simulink model "MicroFSMPCCLACPU1"  (R2024a)
settings: Solver=FixedStepAuto  StartTime=0.0  StopTime=Inf  RelTol=1e-3  EnableMultiTasking=on
values from neighbouring files (symbols this model uses):
  ar = single(round(1/10,3))    [Para_Motor_Micro.m]
  PI_params = mcb.internal.SetControllerParameters(pmsm,inverter,SI_System,T_pwm,Ts,Ts_speed)    [Para_Motor_Micro.m]
  Tabf = round(Tab',3)    [Para_Motor_Micro.m]
  target = mcb_SetProcessorDetails('F28379D',PWM_frequency)    [Para_Motor_Micro.m]
  Ts = T_pwm    (= 3e-05)    [Para_Motor_Micro.m]
  Ts_com = 2*1*Ts    (= 6e-05)    [Para_Motor_Micro.m]
undefined symbols (not defined in the file or in its folder): C28x, codertarget, CPU1, CPU2, Down, dyV, gmax, GPTRIP1SEL, GPTRIP2SEL, inverter, Ls, PWM_Counter_PeriodVel, R, Tab, Tv, Tvz, TZ1, TZ2, ud, Up
libraries: mcbcontrolslib x28, c2802xlib x18, c2837xDlib x13, dsparch4 x6, eeTransforms x5, slpidlib x4, mcbpositiondecoderlib x3, simulink x2, c2806xlib x1, spsabctoAlphaBetaZeroLib x1, c280xlib x1, c2000lib x1
(part 6 of 8)

== matlab function MicroFSMPCCLACPU1/ADC-PWM /Control_System/Closed Loop Control/FS-MPC Sobre muestreo modulado ==
  settings: updateMethod=DISCRETE
  data: I input; Gate output size=3; FEM input size=2; iAref input; iBref input; mode input; Vbus input; J output size=1

function [Gate,J]      = fcn(I,FEM,iAref,iBref,mode,Vbus)


%%%%%Init Parameters%%%%%%%
Ts=single(3.2e-5);
R=single(1) ;
L=single(2.00e-3);
M=(3/7)*L;
Ls=single(L+M);
ud=single(170);
%alphe=single(0.5);
gmax=single(10000);
n=single(3);
moder=mode;

% uAnull=single(0);
% uBnull=single(0);
Div=single(4); %%%%Numero de divisiones 
dy0=single(0.12);
dyV=(1-dy0)/Div;
Tv=dyV*Ts;
Tvz=Ts*(dy0/2+dyV);
%Tp=single(Ts*0.9);
 persistent     Gates Gop jop iA1o iB1o Gop1 jop1 iA2o iB2o Gop2 jop2 Gop3 jop3 iA3o iB3o status1  %tick status1 
  if isempty(Gates)
        Gates=single([0,0,0]');

        Gop=gmax;
        jop=single(1);
        iA1o=single(0);
        iB1o=single(0);

        Gop1=gmax;
        jop1=single(1);
        iA2o=single(0);
        iB2o=single(0);

        Gop2=gmax;
        jop2=single(1);
        iA3o=single(0);
        iB3o=single(0);

        Gop3=gmax;
        jop3=single(1);

     end


%%%%%%Read mesurments%%%%%%%%%%%%
%ud=single(Vbus);
iA=I(1);
iB=I(2);
eA=FEM(1);
eB=FEM(2);

% eA1=FEM1(1);
% eB1=FEM1(2);
% fa=eA/(Ke*w);
% fb=eB/(Ke*w);
% fa1=fa;
% fb1=fb;
% ua=u(1);
% ub=u(2);



 % % %%%7 vectores ordenados ab separados flotando
%  status1=[0,1,0,1,0,1	;
%      1,0,0,0,0,1	;
%  0,0,1,0,0,1	;
%  0,1,1,0,0,0	;
%  0,1,0,0,1,0	;
%  0,0,0,1,1,0	;
%  1,0,0,1,0,0	;];
% 
%  u1=ud*[0	,	0	;
%      1/2	,	sqrt(3)/6 	;
% 0	,	sqrt(3)/3	;
% -1/2	,	sqrt(3)/6 	;
% -1/2	,	-sqrt(3)/6 	;
% 0	,	-sqrt(3)/3	;
% 1/2	,	-sqrt(3)/6 	;
% ];

%%%%%%For loop 3%%%%%%      
% %%%7 vectores ordenados ab tradicionales
%  status1=[1,1,1;
%           1,0,0	;
%           1,1,0;
%           0,1,0;
%            0,1,1	;
%            0,0,1	;
%            1,0,1;
%            ];
% % 
%  u1=ud*[0	,	0	;
%       2/3	,	0	;
%       1/3	,	1/sqrt(3)	;%parece estar aml el vector
%   -1/3	,	1/sqrt(3)	;
%  -2/3	,	0	;
%  -1/3	,	-1/sqrt(3)	;
%   1/3	,	-1/sqrt(3)	;
%   ];


 if mode==1
  u1=ud*[0	,	0	;
2/3	,	0	;
1/3	,	1/sqrt(3)];
elseif mode==2
 
 u1=ud*[0	,	0	;
1/3	,	1/sqrt(3)	;
-1/3	,	1/sqrt(3)	;];   
elseif mode==3

 u1=ud*[0	,	0	;
-1/3	,	1/sqrt(3)	;
-2/3	,	0	;];  
 elseif mode==4
 
 u1=ud*[0	,	0	;
-2/3	,	0	;
-1/3	,	-1/sqrt(3)	;];
 elseif mode==5
  
 u1=ud*[0	,	0	;
-1/3	,	-1/sqrt(3)	;
1/3	,	-1/sqrt(3)	;];
 elseif mode==6
  
 u1=ud*[0	,	0	;
1/3	,	-1/sqrt(3)	;
2/3	,	0	;];

else
   
 u1=ud*[0	,	0	;
2/3	,	0	;
1/3	,	1/sqrt(3)]; 
end

%%%%%%%%FSMPC%%%%%%%%%%%%%%%%%%%%%%%%%%%%%%%%%%%%%

      Gop=gmax;
      jop=single(1);
      Gop1=gmax;
      jop1=single(1);
      Gop2=gmax;
      jop2=single(1);
      Gop3=gmax;
      jop3=single(1);

%%%%%%For n loop N1  %%%%%% 
     for j= 1:n    
  uA1=u1(j,1);
  uB1=u1(j,2);

%%%%%%For loop 3 combinacion de vectores 1%%%%%% 
     iA1= iA + (1/Ls)*(Tv*uA1)- (Tvz/Ls)*(eA+R*iA);
     iB1=iB + (1/Ls)*(Tv*uB1)- (Tvz/Ls)*(eB+R*iB);
     
     G=(iAref-iA1)^2+(iBref-iB1)^2 ; 

          if G<Gop
          Gop=G;
          jop=j;
          iA1o=iA1;
          iB1o=iB1;
   
          end
     end

 %%%%%%For n loop N2  %%%%%% 
  for j1= 1:n    
  uA1=u1(j1,1);
  uB1=u1(j1,2);

%%%%%%For loop 3 combinacion de vectores 1%%%%%% 
     iA1= iA1o + (1/Ls)*(Tv*uA1)- (Tv/Ls)*(eA+R*iA1o);
     iB1=iB1o + (1/Ls)*(Tv*uB1)- (Tv/Ls)*(eB+R*iB1o);
     
     G=(iAref-iA1)^2+(iBref-iB1)^2 ; 

          if G<Gop
          Gop1=G;
          jop1=j1;
          iA2o=iA1;
          iB2o=iB1;
   
          end
  end    


 %%%%%%For n loop N3  %%%%%% 
  for j2= 1:n    
  uA1=u1(j2,1);
  uB1=u1(j2,2);

%%%%%%For loop 3 combinacion de vectores 1%%%%%% 
     iA1= iA2o + (1/Ls)*(Tv*uA1)- (Tv/Ls)*(eA+R*iA2o);
     iB1=iB2o + (1/Ls)*(Tv*uB1)- (Tv/Ls)*(eB+R*iB2o);
     
     G=(iAref-iA1)^2+(iBref-iB1)^2 ; 

          if G<Gop
          Gop2=G;
          jop2=j2;
          iA3o=iA1;
          iB3o=iB1;
   
          end
  end   
  

 %%%%%%For n loop N4  %%%%%% 
  for j3= 1:n    
  uA1=u1(j3,1);
  uB1=u1(j3,2);

%%%%%%For loop 3 combinacion de vectores 1%%%%%% 
     iA1= iA3o + (1/Ls)*(Tv*uA1)- (Tvz/Ls)*(eA+R*iA3o);
     iB1=iB3o + (1/Ls)*(Tv*uB1)- (Tvz/Ls)*(eB+R*iB3o);
     
     G=(iAref-iA1)^2+(iBref-iB1)^2 ; 

          if G<Gop
          Gop3=G;
          jop3=j3;
      
   
          end
  end   

    
%%%%Apply conmutation states%%%%%%%%%%%%%%%%%%%%%%%  


   % Gates=status1(jop,:)';

%To=dyV*((indexv(1,jop)==1)+(indexv(2,jop)==1)+(indexv(3,jop)==1)+(indexv(4,jop)==1))+dy0;
%To=0;
% Ta=dyV*((indexv(1,jop)==2)+(indexv(2,jop)==2)+(indexv(3,jop)==2)+(indexv(4,jop)==2));
% Tb=dyV*((indexv(1,jop)==3)+(indexv(2,jop)==3)+(indexv(3,jop)==3)+(indexv(4,jop)==3));
Ta=dyV*((jop==2)+(jop1==2)+(jop2==2)+(jop3==2));
Tb=dyV*((jop==3)+(jop1==3)+(jop2==3)+(jop3==3));

  TA=(moder==1)*(Tb+Ta)+(moder==6)*(Tb+Ta)+(moder==2)*(Ta)+(moder==5)*(Tb);
  TB=(moder==1)*(Tb)+(moder==2)*(Tb+Ta)+(moder==3)*(Tb+Ta)+(moder==4)*(Ta);
  TC=(moder==6)*(Ta)+(moder==3)*(Tb)+(moder==4)*(Tb+Ta)+(moder==5)*(Tb+Ta);




% TA=(moder==6)*(To+Tb+Ta)+(moder==5)*(To+Tb+Ta)+(moder==1)*(To+Ta)+(moder==2)*(To)+(moder==3)*(To)+(moder==4)*(To+Tb);
% TB=(moder==5)*(To)+(moder==6)*(To+Tb)+(moder==1)*(To+Tb+Ta)+(moder==2)*(To+Tb+Ta)+(moder==3)*(To+Ta)+(moder==4)*(To);
% TC=(moder==5)*(To+Ta)+(moder==6)*(To)+(moder==1)*(To)+(moder==2)*(To+Tb)+(moder==3)*(To+Tb+Ta)+(moder==4)*(To+Tb+Ta);

Gates=[TA,TB,TC]';
J=jop;
Gate=Gates;
%tie=t2;
%jl=jn;
%j=1;




%   TA=(moder==1)*(To+Tb+Ta)+(moder==6)*(To+Tb+Ta)+(moder==2)*(To+Ta)+(moder==3)*(To)+(moder==4)*(To)+(moder==5)*(To+Tb);
% % TA=(moder==6)*(To+Tb+Ta)+(moder==5)*(To+Tb+Ta)+(moder==1)*(To+Ta)+(moder==2)*(To)+(moder==3)*(To)+(moder==4)*(To+Tb);
%   TB=(moder==6)*(To)+(moder==1)*(To+Tb)+(moder==2)*(To+Tb+Ta)+(moder==3)*(To+Tb+Ta)+(moder==4)*(To+Ta)+(moder==5)*(To);
% % TB=(moder==5)*(To)+(moder==6)*(To+Tb)+(moder==1)*(To+Tb+Ta)+(moder==2)*(To+Tb+Ta)+(moder==3)*(To+Ta)+(moder==4)*(To);
%   TC=(moder==6)*(To+Ta)+(moder==1)*(To)+(moder==2)*(To)+(moder==3)*(To+Tb)+(moder==4)*(To+Tb+Ta)+(moder==5)*(To+Tb+Ta);

== matlab function MicroFSMPCCLACPU1/ADC-PWM /Control_System/Closed Loop Control/FS-MPC Sobre muestreo modulado clean ==
  settings: updateMethod=DISCRETE
  data: I input; Gate output size=3; FEM input size=2; iAref input; iBref input; mode input; J output size=1; Ts parameter; R parameter; Ls parameter; ud parameter; gmax parameter; Tv parameter; Tvz parameter; dyV parameter

function [Gate, J]      = fcn(I,FEM,iAref,iBref,mode,Ts, R, Ls, ud, gmax, Tv, Tvz, dyV)


%%%%%Init Parameters%%%%%%%
% Ts=single(2.5e-5);
% %Ts=single(5e-5);
% %Ts=single(3.2e-05);
% R=single(1) ;
% %L=single(9.75e-3);
%  L=single(2.02e-3);
% %L=single(1.45e-3);
%   %L=single(Lp);
%   %L=single(1.85e-3);
%  M=(3/7)*L;
% %Lt=(7/3)*M;
% Ls=single(L+M);
% %Ls=single(L);
% %Ls=single(L);
% %ud=240;
% ud=single(170);

%Kt =single(0.3811);
%T0=Ts*(1);
%Ke=single(0.3455);
%gmax=single(100000);
n=single(3);

% % uAnull=single(0);
% % uBnull=single(0);
% Div=single(4); %%%%Numero de divisiones 
% dy0=single(0.1);
% dyV=(1-dy0)/Div;
% Tv=dyV*Ts;
% Tvz=Ts*(dy0/2+dyV);
%Tp=single(Ts*0.9);
 persistent     Gates Gop jop iA1o iB1o Gop1 jop1 iA2o iB2o Gop2 jop2 Gop3 jop3 iA3o iB3o  %tick status1 
  if isempty(Gates)
        Gates=single([0,0,0]');

        Gop=gmax;
        jop=single(1);
        iA1o=single(0);
        iB1o=single(0);

        Gop1=gmax;
        jop1=single(1);
        iA2o=single(0);
        iB2o=single(0);

        Gop2=gmax;
        jop2=single(1);
        iA3o=single(0);
        iB3o=single(0);

        Gop3=gmax;
        jop3=single(1);


     end


%%%%%%Read mesurments%%%%%%%%%%%%
%ud=single(Vbus);

iA=I(1);
iB=I(2);
eA=FEM(1);
eB=FEM(2);
moder=mode;



 if mode==1
 u1=ud*[0	,	0	;
2/3	,	0	;
1/3	,	1/sqrt(3)];
elseif mode==2
 
 u1=ud*[0	,	0	;
1/3	,	1/sqrt(3)	;
-1/3	,	1/sqrt(3)	;];   
elseif mode==3
   
 u1=ud*[0	,	0	;
-1/3	,	1/sqrt(3)	;
-2/3	,	0	;];  
 elseif mode==4
  
 u1=ud*[0	,	0	;
-2/3	,	0	;
-1/3	,	-1/sqrt(3)	;];
 elseif mode==5
   
 u1=ud*[0	,	0	;
-1/3	,	-1/sqrt(3)	;
1/3	,	-1/sqrt(3)	;];
 elseif mode==6
   
 u1=ud*[0	,	0	;
1/3	,	-1/sqrt(3)	;
2/3	,	0	;];

else
 
 u1=ud*[0	,	0	;
2/3	,	0	;
1/3	,	1/sqrt(3)]; 
end

%%%%%%%%FSMPC%%%%%%%%%%%%%%%%%%%%%%%%%%%%%%%%%%%%%

      Gop=gmax;
      jop=single(1);
      Gop1=gmax;
      jop1=single(1);
      Gop2=gmax;
      jop2=single(1);
      Gop3=gmax;
      jop3=single(1);

%%%%%%For n loop N1  %%%%%% 
     for j= 1:n    
  uA1=u1(j,1);
  uB1=u1(j,2);

%%%%%%For loop 3 combinacion de vectores 1%%%%%% 
     iA1= iA + (1/Ls)*(Tv*uA1)- (Tvz/Ls)*(eA+R*iA);
     iB1=iB + (1/Ls)*(Tv*uB1)- (Tvz/Ls)*(eB+R*iB);
     
     G=(iAref-iA1)^2+(iBref-iB1)^2 ; 

          if G<Gop
          Gop=G;
          jop=j;
          iA1o=iA1;
          iB1o=iB1;
   
          end
     end

 %%%%%%For n loop N2  %%%%%% 
  for j1= 1:n    
  uA1=u1(j1,1);
  uB1=u1(j1,2);

%%%%%%For loop 3 combinacion de vectores 1%%%%%% 
     iA1= iA1o + (1/Ls)*(Tv*uA1)- (Tv/Ls)*(eA+R*iA1o);
     iB1=iB1o + (1/Ls)*(Tv*uB1)- (Tv/Ls)*(eB+R*iB1o);
     
     G=(iAref-iA1)^2+(iBref-iB1)^2 ; 

          if G<Gop
          Gop1=G;
          jop1=j1;
          iA2o=iA1;
          iB2o=iB1;
   
          end
  end    


 %%%%%%For n loop N3  %%%%%% 
  for j2= 1:n    
  uA1=u1(j2,1);
  uB1=u1(j2,2);

%%%%%%For loop 3 combinacion de vectores 1%%%%%% 
     iA1= iA2o + (1/Ls)*(Tv*uA1)- (Tv/Ls)*(eA+R*iA2o);
     iB1=iB2o + (1/Ls)*(Tv*uB1)- (Tv/Ls)*(eB+R*iB2o);
     
     G=(iAref-iA1)^2+(iBref-iB1)^2 ; 

          if G<Gop
          Gop2=G;
          jop2=j2;
          iA3o=iA1;
          iB3o=iB1;
   
          end
  end   
  

 %%%%%%For n loop N4  %%%%%% 
  for j3= 1:n    
  uA1=u1(j3,1);
  uB1=u1(j3,2);

%%%%%%For loop 3 combinacion de vectores 1%%%%%% 
     iA1= iA3o + (1/Ls)*(Tv*uA1)- (Tvz/Ls)*(eA+R*iA3o);
     iB1=iB3o + (1/Ls)*(Tv*uB1)- (Tvz/Ls)*(eB+R*iB3o);
     
     G=(iAref-iA1)^2+(iBref-iB1)^2 ; 

          if G<Gop
          Gop3=G;
          jop3=j3;
      
   
          end
  end   

    
%%%%Apply conmutation states%%%%%%%%%%%%%%%%%%%%%%%  


Ta=dyV*((jop==2)+(jop1==2)+(jop2==2)+(jop3==2));
Tb=dyV*((jop==3)+(jop1==3)+(jop2==3)+(jop3==3));

  TA=(moder==1)*(Tb+Ta)+(moder==6)*(Tb+Ta)+(moder==2)*(Ta)+(moder==5)*(Tb);
  TB=(moder==1)*(Tb)+(moder==2)*(Tb+Ta)+(moder==3)*(Tb+Ta)+(moder==4)*(Ta);
  TC=(moder==6)*(Ta)+(moder==3)*(Tb)+(moder==4)*(Tb+Ta)+(moder==5)*(Tb+Ta);


Gates=[TA,TB,TC]';
J=jop;
Gate=Gates;

== matlab function MicroFSMPCCLACPU1/ADC-PWM /Control_System/Closed Loop Control/FS-MPC opt tiempo complex Clean ==
  settings: updateMethod=DISCRETE
  data: I input; Gate output size=3; FEM input size=2; iAref input; iBref input; J output size=1; mode input; moder input

function [Gate,J]      = fcn(I,FEM,iAref,iBref,mode,moder)


%%%%%Init Parameters%%%%%%%
Ts=single(2.5e-5);
R=single(1) ;
L=single(1.85e-3);
M=(3/7)*L;
Ls=single(L+M);
ud=single(170);
alphe=single(0.5);
gmax=single(10000);
n=single(3);
nk=single(3);


 persistent     Gates Gop jop  Trop Tr  status1
  if isempty(Gates)
        Gates=single([0,0,0]');
        Gop=gmax;
        jop=single(1);
        Tr=single(0);
        Trop=single(0);

status1=[
 1,1,0;
 0,1,0;
 0,0,0;]; 
     end


%%%%%%Read mesurments%%%%%%%%%%%%
iA=I(1);
iB=I(2);
eA=FEM(1);
eB=FEM(2);


%%%%Moded
%  if mode==1
%  status1=[0,0,0;
%  1,0,0	;
% 1,1,0;];   
%  u1=ud*[0	,	0	;
% 2/3	,	0	;
% 1/3	,	1/sqrt(3)];
% elseif mode==2
%  status1=[0,0,0;
% 1,1,0	;
% 0,1,0	;];   
%  u1=ud*[0	,	0	;
% 1/3	,	1/sqrt(3)	;
% -1/3	,	1/sqrt(3)	;];   
% elseif mode==3
%  status1=[0,0,0;
% 0,1,0	;
% 0,1,1	;];   
%  u1=ud*[0	,	0	;
% -1/3	,	1/sqrt(3)	;
% -2/3	,	0	;];  
%  elseif mode==4
%  status1=[0,0,0;
%  0,1,1	;
% 0,0,1	;];   
%  u1=ud*[0	,	0	;
% -2/3	,	0	;
% -1/3	,	-1/sqrt(3)	;];
%  elseif mode==5
%  status1=[0,0,0;
%  0,0,1	;
% 1,0,1	;];   
%  u1=ud*[0	,	0	;
% -1/3	,	-1/sqrt(3)	;
% 1/3	,	-1/sqrt(3)	;];
%  elseif mode==6
%  status1=[0,0,0
% 1,0,1	;
%  1,0,0	;];   
%  u1=ud*[0	,	0	;
% 1/3	,	-1/sqrt(3)	;
% 2/3	,	0	;];
% 
% else
%  status1=[0,0,0;
%  1,0,0	;
% 1,1,0;];   
%  u1=ud*[0	,	0	;
% 2/3	,	0	;
% 1/3	,	1/sqrt(3)]; 
% end

%%%13 vectores totales, 12 modes
 if mode==1 %%%%V0,V1,V12
 u1=ud*[2/3	,	0	;
1/2	,	1/(2*sqrt(3));
0	,	0	;];
elseif mode==2 %%%%V0,V12,V2
 u1=ud*[1/2	,	1/(2*sqrt(3))	;
1/3	,	1/sqrt(3);
0	,	0	;];

elseif mode==3
  u1=ud*[1/3	,	1/sqrt(3)	;
0	,	1/sqrt(3)	;
0	,	0	;];   
  elseif mode==4
  u1=ud*[0	,	1/sqrt(3)	;
-1/3	,	1/sqrt(3)	;
0	,	0	;]; 


elseif mode==5
 u1=ud*[-1/3	,	1/sqrt(3)	;
-1/2	,	1/(2*sqrt(3))	;
0	,	0	;];  

elseif mode==6
 u1=ud*[-1/2	,	1/(2*sqrt(3))	;
-2/3	,	0	;
0	,	0	;];  

 elseif mode==7
 u1=ud*[-2/3	,	0	;
-1/2	,	-1/(2*sqrt(3));
0	,	0	;];

  elseif mode==8
 u1=ud*[-1/2	,	-1/(2*sqrt(3))	;
-1/3	,	-1/sqrt(3)	;
0	,	0	;];


 elseif mode==9
 u1=ud*[
-1/3	,	-1/sqrt(3)	;
0	,	-1/sqrt(3)	;
0	,	0	;];

  elseif mode==10
 u1=ud*[
0	,	-1/sqrt(3)	;
1/3	,	-1/sqrt(3)	;
0	,	0	;];


 elseif mode==11
 u1=ud*[
1/3	,	-1/sqrt(3)	;
1/2	,	-1/(2*sqrt(3))	;
0	,	0	;];

  elseif mode==12
 u1=ud*[
1/2	,	-1/(2*sqrt(3))	;
2/3	,	0	;
0	,	0	;];

else
 
 u1=ud*[
2/3	,	0	;
1/3	,	1/sqrt(3);
0	,	0	;]; 
end
%%%%%%%%FSMPC%%%%%%%%%%%%%%%%%%%%%%%%%%%%%%%%%%%%%

      Gop=gmax;
      jop=single(1);
       ar=single(0.9/7);
%%%%%%For n loop N1  %%%%%% 
for p= 1:nk

    if p==1
        n=single(3);
    else
        n=single(2);
    end    
    Tr1=ar*(2*p);

%%%%%%%%%%%%%%%%%%%%%%%%%%%%%%%%%%%%%%%%%%%%%%%%%%
     for j= 1:n    
     uA1=u1((j),1);
     uB1=u1((j),2);
%%%%%%For loop %%%%%%%%%%%%%%%%%%%%%%%%%%%%%%%%% 
     iA1= iA + (1/Ls)*(Tr1*Ts*uA1)- (Ts/Ls)*(eA+R*iA);
     iB1=iB + (1/Ls)*(Tr1*Ts*uB1)- (Ts/Ls)*(eB+R*iB);
     G=(iAref-iA1)^2+(iBref-iB1)^2 ; 
     % G=abs(iAref-iA1)+abs(iBref-iB1) ; 
          if G<Gop
          Gop=G;
          jop=j;
          Tr=Tr1;
          end
     end
end
%%%%%%%%%%%%%%%%%%%%%%%%%%%%%%%%%%%%%%%%%%%%%%%%%

%%%%Segunda vuelta%%%%%
     uA1=u1((jop),1);
     uB1=u1((jop),2);
%%%%%%%%%%%%%%%%%%%%%%%%%%%%%%%%%%%%%%%%%%%%%%%%%%
%      for p= 1:2    
% %%%%%%For loop %%%%%%%%%%%%%%%%%%%%%%%%%%%%%%%%% 
%     if p==1
%      Trop=Tr;
%      Tr1=Trop-ar; 
%      else
%      Tr1=Trop+ar;
%     end
  for j= 1:2 
     if j==1
     Trop=Tr;
     Tr1=Trop-ar; 
     else
     Tr1=Trop+ar;
    end
%      uA1=u1((j),1);
%      uB1=u1((j),2);
     iA1= iA + (1/Ls)*(Tr1*Ts*uA1)- (Ts/Ls)*(eA+R*iA);
     iB1=iB + (1/Ls)*(Tr1*Ts*uB1)- (Ts/Ls)*(eB+R*iB);
     G=(iAref-iA1)^2+(iBref-iB1)^2 ; 
       %G=abs(iAref-iA1)+abs(iBref-iB1) ; 
          if G<Gop
          Gop=G;
          %jop=single(j);
          Tr=Tr1;
          end
  end
%      end

%%%%%%%%%%%%%%%%%%%%%%%%%%%%%%%%%%%%%%%%%%%%%%%%%
    
%%%%Apply conmutation states%%%%%%%%%%%%%%%%%%%%%%%  


%%%%%%12 vectores
if mod(mode,2)==1
a1=single(1);
a2=alphe;
a3=single(0);
a4=alphe;
else
a1=alphe;
a2=single(0);
a3=alphe;
a4=single(1);
end
% %%%%%%%%%%%%
Ta=Tr*(a1*(jop==1)+a2*(jop==2));
Tb=Tr*(a3*(jop==1)+a4*(jop==2));

% Ta=Tr*((jop==1));
% Tb=Tr*((jop==2));


TA=(moder==1)*(Tb+Ta)+(moder==6)*(Tb+Ta)+(moder==2)*(Ta)+(moder==5)*(Tb);
  TB=(moder==1)*(Tb)+(moder==2)*(Tb+Ta)+(moder==3)*(Tb+Ta)+(moder==4)*(Ta);
  TC=(moder==6)*(Ta)+(moder==3)*(Tb)+(moder==4)*(Tb+Ta)+(moder==5)*(Tb+Ta);

Gates=[TA,TB,TC]';
J=jop;
Gate=Gates;

== matlab function MicroFSMPCCLACPU1/ADC-PWM /Control_System/Closed Loop Control/FS-MPC opt tiempo complex Clean 1for ==
  settings: updateMethod=DISCRETE
  data: I input single size=2; Gate output single size=3; FEM input single size=2; iAref input single size=1; iBref input single size=1; J output single size=1; mode input single size=1; moder input single size=1

function [Gate,J]      = fcn(I,FEM,iAref,iBref,mode,moder)


%%%%%Init Parameters%%%%%%%
Ts=single(2.5e-5);
R=single(1) ;
L=single(2.05e-3);
M=(3/7)*L;
Ls=single(L+M);
ud=single(170);
alphe=single(0.5);
gmax=single(10000);
n=single(7);
%nk=single(3);


 persistent     Gates Gop jop  Trop Tr  status1
  if isempty(Gates)
        Gates=single([0,0,0]');
        Gop=gmax;
        jop=single(1);
        Tr=single(0);
        Trop=single(0);

% status1=[
%  1,1,0;
%  0,1,0;
%  0,0,0;]; 
     end


%%%%%%Read mesurments%%%%%%%%%%%%
iA=I(1);
iB=I(2);
eA=FEM(1);
eB=FEM(2);


%%%%Moded
%  if mode==1
%  status1=[0,0,0;
%  1,0,0	;
% 1,1,0;];   
%  u1=ud*[0	,	0	;
% 2/3	,	0	;
% 1/3	,	1/sqrt(3)];
% elseif mode==2
%  status1=[0,0,0;
% 1,1,0	;
% 0,1,0	;];   
%  u1=ud*[0	,	0	;
% 1/3	,	1/sqrt(3)	;
% -1/3	,	1/sqrt(3)	;];   
% elseif mode==3
%  status1=[0,0,0;
% 0,1,0	;
% 0,1,1	;];   
%  u1=ud*[0	,	0	;
% -1/3	,	1/sqrt(3)	;
% -2/3	,	0	;];  
%  elseif mode==4
%  status1=[0,0,0;
%  0,1,1	;
% 0,0,1	;];   
%  u1=ud*[0	,	0	;
% -2/3	,	0	;
% -1/3	,	-1/sqrt(3)	;];
%  elseif mode==5
%  status1=[0,0,0;
%  0,0,1	;
% 1,0,1	;];   
%  u1=ud*[0	,	0	;
% -1/3	,	-1/sqrt(3)	;
% 1/3	,	-1/sqrt(3)	;];
%  elseif mode==6
%  status1=[0,0,0
% 1,0,1	;
%  1,0,0	;];   
%  u1=ud*[0	,	0	;
% 1/3	,	-1/sqrt(3)	;
% 2/3	,	0	;];
% 
% else
%  status1=[0,0,0;
%  1,0,0	;
% 1,1,0;];   
%  u1=ud*[0	,	0	;
% 2/3	,	0	;
% 1/3	,	1/sqrt(3)]; 
% end

%%%13 vectores totales, 12 modes
 if mode==1 %%%%V0,V1,V12
 u1=ud*[2/3	,	0	;
1/2	,	1/(2*sqrt(3));
0	,	0	;];
elseif mode==2 %%%%V0,V12,V2
 u1=ud*[1/2	,	1/(2*sqrt(3))	;
1/3	,	1/sqrt(3);
0	,	0	;];

elseif mode==3
  u1=ud*[1/3	,	1/sqrt(3)	;
0	,	1/sqrt(3)	;
0	,	0	;];   
  elseif mode==4
  u1=ud*[0	,	1/sqrt(3)	;
-1/3	,	1/sqrt(3)	;
0	,	0	;]; 


elseif mode==5
 u1=ud*[-1/3	,	1/sqrt(3)	;
-1/2	,	1/(2*sqrt(3))	;
0	,	0	;];  

elseif mode==6
 u1=ud*[-1/2	,	1/(2*sqrt(3))	;
-2/3	,	0	;
0	,	0	;];  

 elseif mode==7
 u1=ud*[-2/3	,	0	;
-1/2	,	-1/(2*sqrt(3));
0	,	0	;];

  elseif mode==8
 u1=ud*[-1/2	,	-1/(2*sqrt(3))	;
-1/3	,	-1/sqrt(3)	;
0	,	0	;];


 elseif mode==9
 u1=ud*[
-1/3	,	-1/sqrt(3)	;
0	,	-1/sqrt(3)	;
0	,	0	;];

  elseif mode==10
 u1=ud*[
0	,	-1/sqrt(3)	;
1/3	,	-1/sqrt(3)	;
0	,	0	;];


 elseif mode==11
 u1=ud*[
1/3	,	-1/sqrt(3)	;
1/2	,	-1/(2*sqrt(3))	;
0	,	0	;];

  elseif mode==12
 u1=ud*[
1/2	,	-1/(2*sqrt(3))	;
2/3	,	0	;
0	,	0	;];

else
 
 u1=ud*[
2/3	,	0	;
1/3	,	1/sqrt(3);
0	,	0	;]; 
end
%%%%%%%%FSMPC%%%%%%%%%%%%%%%%%%%%%%%%%%%%%%%%%%%%%

      Gop=gmax;
      jop=single(1);
       ar=single(0.9/7);
%%%%%%For n loop N1  %%%%%% 
% for p= 1:nk
% 
%     if p==1
%         n=single(3);
%     else
%         n=single(2);
%     end    
%     Tr1=ar*(2*p);

%%%%%%%%%%%%%%%%%%%%%%%%%%%%%%%%%%%%%%%%%%%%%%%%%%
     for j= 1:n    

switch j
    case 1
        Tr1=ar*single(2);
        v=single(1);
    case 2
        Tr1=ar*single(2);
        v=single(2);
     case 3
        Tr1=ar*single(2);
        v=single(3) ; 

    case 4
        Tr1=ar*single(4);
        v=single(1);
    case 5
        Tr1=ar*single(4);
        v=single(2);
    case 6
        Tr1=ar*single(6);
        v=single(1);     
    case 7
        Tr1=ar*single(6);
        v=single(2) ; 
       
    otherwise
        Tr1=ar*single(2);
        v=single(1);
end

if n<=7
v=single(2-mod(n,2));
else
v=single(3);
end
if n<=2
    Tr1=ar*single(2);
elseif n<=4
  Tr1=ar*single(4);
else
     Tr1=ar*single(6);
end



     uA1=u1((v),1);
     uB1=u1((v),2);
%%%%%%For loop %%%%%%%%%%%%%%%%%%%%%%%%%%%%%%%%% 
%      iA1= iA + (1/Ls)*(Tr1*Ts*uA1)- (Ts/Ls)*(eA+R*iA);
%      iB1=iB + (1/Ls)*(Tr1*Ts*uB1)- (Ts/Ls)*(eB+R*iB);
     iA1= (1/(Ts*R+Ls))*(Ls*iA+(Tr1*Ts*uA1)- Ts*eA);
     iB1=(1/(Ts*R+Ls))*(Ls*iB+(Tr1*Ts*uB1)- Ts*eB);
     G=(iAref-iA1)^2+(iBref-iB1)^2 ; 
     % G=abs(iAref-iA1)+abs(iBref-iB1) ; 
          if G<Gop
          Gop=G;
          jop=v;
          Tr=Tr1;
          end
     end
%end
%%%%%%%%%%%%%%%%%%%%%%%%%%%%%%%%%%%%%%%%%%%%%%%%%

% %%%%Segunda vuelta%%%%%
%      uA1=u1((jop),1);
%      uB1=u1((jop),2);
% %%%%%%%%%%%%%%%%%%%%%%%%%%%%%%%%%%%%%%%%%%%%%%%%%%
% %      for p= 1:2    
% % %%%%%%For loop %%%%%%%%%%%%%%%%%%%%%%%%%%%%%%%%% 
% %     if p==1
% %      Trop=Tr;
% %      Tr1=Trop-ar; 
% %      else
% %      Tr1=Trop+ar;
% %     end
%   for j= 1:2 
%      if j==1
%      Trop=Tr;
%      Tr1=Trop-ar; 
%      else
%      Tr1=Trop+ar;
%     end
% %      uA1=u1((j),1);
% %      uB1=u1((j),2);
%      iA1= iA + (1/Ls)*(Tr1*Ts*uA1)- (Ts/Ls)*(eA+R*iA);
%      iB1=iB + (1/Ls)*(Tr1*Ts*uB1)- (Ts/Ls)*(eB+R*iB);
%      G=(iAref-iA1)^2+(iBref-iB1)^2 ; 
%        %G=abs(iAref-iA1)+abs(iBref-iB1) ; 
%           if G<Gop
%           Gop=G;
%           Tr=Tr1;
%           end
%   end
   %  end

%%%%%%%%%%%%%%%%%%%%%%%%%%%%%%%%%%%%%%%%%%%%%%%%%
    
%%%%Apply conmutation states%%%%%%%%%%%%%%%%%%%%%%%  


%%%%%%12 vectores
if mod(mode,2)==1
a1=single(1);
a2=alphe;
a3=single(0);
a4=alphe;
else
a1=alphe;
a2=single(0);
a3=alphe;
a4=single(1);
end
% %%%%%%%%%%%%
Ta=Tr*(a1*(jop==1)+a2*(jop==2));
Tb=Tr*(a3*(jop==1)+a4*(jop==2));

% Ta=Tr*((jop==1));
% Tb=Tr*((jop==2));


TA=(moder==1)*(Tb+Ta)+(moder==6)*(Tb+Ta)+(moder==2)*(Ta)+(moder==5)*(Tb);
  TB=(moder==1)*(Tb)+(moder==2)*(Tb+Ta)+(moder==3)*(Tb+Ta)+(moder==4)*(Ta);
  TC=(moder==6)*(Ta)+(moder==3)*(Tb)+(moder==4)*(Tb+Ta)+(moder==5)*(Tb+Ta);

Gates=[TA,TB,TC]';
J=jop;
Gate=Gates;

== matlab function MicroFSMPCCLACPU1/ADC-PWM /Control_System/Closed Loop Control/FS-MPC opt tiempo complex Clean 1for Table ==
  settings: updateMethod=DISCRETE
  data: I input single size=2; Gate output single size=3; FEM input single size=2; iAref input single size=1; iBref input single size=1; J output single size=1; mode input single size=1; Tabf parameter single; ar parameter; Ts parameter; R parameter; Ls parameter; ud parameter; gmax parameter

function [Gate,J]      = fcn(I,FEM,iAref,iBref,mode, Tabf,ar,Ts, R, Ls,ud, gmax )


%%%%%Init Parameters%%%%%%%
% 
% Ts=single(2.5e-5);
% R=single(1) ;
% L=single(2.02e-3);
% %L=single(Lp);
% M=(3/7)*L;
% Ls=single(L+M);
%ud=single(170);
%gmax=single(10000);
n=single(7+4);
moder=mode;
Tabfn=single([0,0;0,0;0,0;0,0]);

 persistent     Gates Gop jop  Tr Tao Tbo  
  if isempty(Gates)
        Gates=single([0,0,0]');
        Gop=gmax;
        jop=single(1);
        Tr=single(0);
        Tao=single(0);
Tbo=single(0);

     end


%%%%%%Read mesurments%%%%%%%%%%%%
iA=I(1);
iB=I(2);
eA=FEM(1);
eB=FEM(2);




% % %%%7 Vectores totales
 if mode==1
 u1=ud*[2/3	,	0	;
1/3	,	1/sqrt(3);
0	,	0	;];
elseif mode==2
 u1=ud*[1/3	,	1/sqrt(3)	;
-1/3	,	1/sqrt(3)	;
0	,	0	;];   
elseif mode==3
 u1=ud*[-1/3	,	1/sqrt(3)	;
-2/3	,	0	;
0	,	0	;];  
 elseif mode==4
 u1=ud*[-2/3	,	0	;
-1/3	,	-1/sqrt(3)	;
0	,	0	;];
 elseif mode==5
 u1=ud*[-1/3	,	-1/sqrt(3)	;
1/3	,	-1/sqrt(3)	;
0	,	0	;];
 elseif mode==6
 u1=ud*[1/3	,	-1/sqrt(3)	;
2/3	,	0	;
0	,	0	;];
else
 u1=ud*[2/3	,	0	;
1/3	,	1/sqrt(3);
0	,	0	;]; 
end
%%%%%%%




%%%%%%%%FSMPC%%%%%%%%%%%%%%%%%%%%%%%%%%%%%%%%%%%%%

      Gop=gmax;
      jop=single(1);
     uA1=u1(1,1);
     uB1=u1(1,2);
     uA2=u1(2,1);
     uB2=u1(2,2);
     %  ar=single(0.9/7);
%%%%%%For n loop N1  %%%%%% 





   

%%%%%%For n loop  %%%%%% 
     for j= 1:n    
   
if j==8
t1=Tr+ar;
t2=Tr-ar;
Tabfn=single([t1,0;0,t1;t2,0;0,t2]);
end




   if j<=n-4      
    T1=Tabf(j,1);
    T2=Tabf(j,2);
   else
    T1=Tabfn(j-7,1);
    T2=Tabfn(j-7,2);

   end


   uA=(T1*uA1 + T2*uA2);
   uB=(T1*uB1 + T2*uB2);

%     for j= 1:n    


% if j<=6
% v=single(2-mod(j,2));
% else
% v=single(3);
% end
% if j<=2
%     Tr1=ar*single(2);
% elseif j<=4
%   Tr1=ar*single(4);
% %   elseif j<=6
% %   Tr1=ar*single(6);
% else
%     % Tr1=ar*single(8);
%       Tr1=ar*single(6);
% end
% 
% 
%      uA1=u1((v),1);
%      uB1=u1((v),2);




     
%%%%%%For loop %%%%%%%%%%%%%%%%%%%%%%%%%%%%%%%%% 
     iA1= iA + (1/Ls)*(Ts*uA)- (Ts/Ls)*(eA+R*iA);
     iB1=iB + (1/Ls)*(Ts*uB)- (Ts/Ls)*(eB+R*iB);
%      iA1= (1/(Ts*R+Ls))*(Ls*iA+(Tr1*Ts*uA1)- Ts*eA);
%      iB1=(1/(Ts*R+Ls))*(Ls*iB+(Tr1*Ts*uB1)- Ts*eB);
     G=(iAref-iA1)^2+(iBref-iB1)^2 ; 
     % G=abs(iAref-iA1)+abs(iBref-iB1) ; 
          if G<Gop
          Gop=G;
          %jop=j;
          Tr=T1+T2;
          Tao=T1;
          Tbo=T2;
          end
     end
%end
%%%%%%%%%%%%%%%%%%%%%%%%%%%%%%%%%%%%%%%%%%%%%%%%%

% %%%%Segunda vuelta%%%%%
%      uA1=u1((jop),1);
%      uB1=u1((jop),2);
% % %%%%%%%%%%%%%%%%%%%%%%%%%%%%%%%%%%%%%%%%%%%%%%%%%%
% % %      for p= 1:2    
% % % %%%%%%For loop %%%%%%%%%%%%%%%%%%%%%%%%%%%%%%%%% 
% % %     if p==1
% % %      Trop=Tr;
% % %      Tr1=Trop-ar; 
% % %      else
% % %      Tr1=Trop+ar;
% % %     end
%   for j= 1:2 
%      if j==1
%      Trop=Tr;
%      Tr1=Trop-ar; 
%      else
%      Tr1=Trop+ar;
%     end
% %      uA1=u1((j),1);
% %      uB1=u1((j),2);
%      iA1= iA + (1/Ls)*(Tr1*Ts*uA1)- (Ts/Ls)*(eA+R*iA);
%      iB1=iB + (1/Ls)*(Tr1*Ts*uB1)- (Ts/Ls)*(eB+R*iB);
%      G=(iAref-iA1)^2+(iBref-iB1)^2 ; 
%        %G=abs(iAref-iA1)+abs(iBref-iB1) ; 
%           if G<Gop
%           Gop=G;
%           Tr=Tr1;
%           end
%   end
 %   end

%%%%%%%%%%%%%%%%%%%%%%%%%%%%%%%%%%%%%%%%%%%%%%%%%
    
%%%%Apply conmutation states%%%%%%%%%%%%%%%%%%%%%%%  


%%%%%%12 vectores
% if mod(mode,2)==1
% a1=single(1);
% a2=alphe;
% a3=single(0);
% a4=alphe;
% else
% a1=alphe;
% a2=single(0);
% a3=alphe;
% a4=single(1);
% end
% %%%%%%%%%%%%
% Ta=Tr*(a1*(jop==1)+a2*(jop==2));
% Tb=Tr*(a3*(jop==1)+a4*(jop==2));

% Ta=Tr*((jop==1));
% Tb=Tr*((jop==2));
% Ta=Tabf(jop,1);
% Tb=Tabf(jop,2);

Ta=Tao;
Tb=Tbo;


TA=(moder==1)*(Tb+Ta)+(moder==6)*(Tb+Ta)+(moder==2)*(Ta)+(moder==5)*(Tb);
TB=(moder==1)*(Tb)+(moder==2)*(Tb+Ta)+(moder==3)*(Tb+Ta)+(moder==4)*(Ta);
TC=(moder==6)*(Ta)+(moder==3)*(Tb)+(moder==4)*(Tb+Ta)+(moder==5)*(Tb+Ta);

Gates=[TA,TB,TC]';
J=jop;
Gate=Gates;

== matlab function MicroFSMPCCLACPU1/ADC-PWM /Control_System/Closed Loop Control/FS-MPC opt tiempo complex Clean 1for Table1 ==
  settings: updateMethod=DISCRETE
  data: I input single size=2; Gate output single size=3; FEM input single size=2; iAref input single size=1; iBref input single size=1; J output single size=1; mode input single size=1; Tabf parameter single; ar parameter; Ts parameter; R parameter; Ls parameter; ud parameter; gmax parameter

function [Gate,J]      = fcn(I,FEM,iAref,iBref,mode, Tabf,ar,Ts, R, Ls,ud, gmax )


%%%%%Init Parameters%%%%%%%
% 
% Ts=single(2.5e-5);
% R=single(1) ;
% L=single(2.02e-3);
% %L=single(Lp);
% M=(3/7)*L;
% Ls=single(L+M);
%ud=single(170);
%gmax=single(10000);
n=single(11);
moder=mode;
%Tabfn=single([0,0;0,0;0,0;0,0]);
p1=single(0);
p2=single(0);

 persistent     Gates Gop jop  Tr Tao Tbo  
  if isempty(Gates)
        Gates=single([0,0,0]');
        Gop=gmax;
        jop=single(1);
        Tr=single(0);
        Tao=single(0);
Tbo=single(0);

     end


%%%%%%Read mesurments%%%%%%%%%%%%
iA=I(1);
iB=I(2);
eA=FEM(1);
eB=FEM(2);




% % %%%7 Vectores totales
 if mode==1
 u1=ud*[2/3	,	0	;
1/3	,	1/sqrt(3);
0	,	0	;];
elseif mode==2
 u1=ud*[1/3	,	1/sqrt(3)	;
-1/3	,	1/sqrt(3)	;
0	,	0	;];   
elseif mode==3
 u1=ud*[-1/3	,	1/sqrt(3)	;
-2/3	,	0	;
0	,	0	;];  
 elseif mode==4
 u1=ud*[-2/3	,	0	;
-1/3	,	-1/sqrt(3)	;
0	,	0	;];
 elseif mode==5
 u1=ud*[-1/3	,	-1/sqrt(3)	;
1/3	,	-1/sqrt(3)	;
0	,	0	;];
 elseif mode==6
 u1=ud*[1/3	,	-1/sqrt(3)	;
2/3	,	0	;
0	,	0	;];
else
 u1=ud*[2/3	,	0	;
1/3	,	1/sqrt(3);
0	,	0	;]; 
end
%%%%%%%




%%%%%%%%FSMPC%%%%%%%%%%%%%%%%%%%%%%%%%%%%%%%%%%%%%

      Gop=gmax;
      jop=single(1);
     %  ar=single(0.9/7);
%%%%%%For n loop N1  %%%%%% 





     uA1=u1(1,1);
     uB1=u1(1,2);
     uA2=u1(2,1);
     uB2=u1(2,2);

%%%%%%For n loop  %%%%%% 
     for j= 1:n    
   
if j==7
p1=Tr+ar;
p2=Tr-ar;
end

   if j<=n-5      
    T1=Tabf(j,1);
    T2=Tabf(j,2);
   elseif j<=n-3  
    T1=p1*Tabf(j,1);
    T2=p1*Tabf(j,2);
   else
    T1=p2*Tabf(j,1);
    T2=p2*Tabf(j,2);
   end


   uA=(T1*uA1 + T2*uA2);
   uB=(T1*uB1 + T2*uB2);
     
%%%%%%For loop %%%%%%%%%%%%%%%%%%%%%%%%%%%%%%%%% 
     iA1= iA + (1/Ls)*(Ts*uA)- (Ts/Ls)*(eA+R*iA);
     iB1=iB + (1/Ls)*(Ts*uB)- (Ts/Ls)*(eB+R*iB);

     G=(iAref-iA1)^2+(iBref-iB1)^2 ; 
     % G=abs(iAref-iA1)+abs(iBref-iB1) ; 
          if G<Gop
          Gop=G;
          %jop=j;
          Tr=T1+T2;
          Tao=T1;
          Tbo=T2;
          end
     end
%end
%%%%%%%%%%%%%%%%%%%%%%%%%%%%%%%%%%%%%%%%%%%%%%%%%

% %%%%Segunda vuelta%%%%%

% 
%  for j= 1:nk  
% 
%      iA1= iA + (1/Ls)*(Ts*uA)- (Ts/Ls)*(eA+R*iA);
%      iB1=iB + (1/Ls)*(Ts*uB)- (Ts/Ls)*(eB+R*iB);
% 
%      G=(iAref-iA1)^2+(iBref-iB1)^2 ; 
% 
%           if G<Gop
%           Gop=G;
%           Tao=T1;
%           Tbo=T2;
%           end
%  end







%%%%%%%%%%%%%%%%%%%%%%%%%%%%%%%%
% %%%%Segunda vuelta%%%%%
%      uA1=u1((jop),1);
%      uB1=u1((jop),2);
% % %%%%%%%%%%%%%%%%%%%%%%%%%%%%%%%%%%%%%%%%%%%%%%%%%%
% % %      for p= 1:2    
% % % %%%%%%For loop %%%%%%%%%%%%%%%%%%%%%%%%%%%%%%%%% 
% % %     if p==1
% % %      Trop=Tr;
% % %      Tr1=Trop-ar; 
% % %      else
% % %      Tr1=Trop+ar;
% % %     end
%   for j= 1:2 
%      if j==1
%      Trop=Tr;
%      Tr1=Trop-ar; 
%      else
%      Tr1=Trop+ar;
%     end
% %      uA1=u1((j),1);
% %      uB1=u1((j),2);
%      iA1= iA + (1/Ls)*(Tr1*Ts*uA1)- (Ts/Ls)*(eA+R*iA);
%      iB1=iB + (1/Ls)*(Tr1*Ts*uB1)- (Ts/Ls)*(eB+R*iB);
%      G=(iAref-iA1)^2+(iBref-iB1)^2 ; 
%        %G=abs(iAref-iA1)+abs(iBref-iB1) ; 
%           if G<Gop
%           Gop=G;
%           Tr=Tr1;
%           end
%   end
 %   end

%%%%%%%%%%%%%%%%%%%%%%%%%%%%%%%%%%%%%%%%%%%%%%%%%
    
%%%%Apply conmutation states%%%%%%%%%%%%%%%%%%%%%%%  


%%%%%%12 vectores
% if mod(mode,2)==1
% a1=single(1);
% a2=alphe;
% a3=single(0);
% a4=alphe;
% else
% a1=alphe;
% a2=single(0);
% a3=alphe;
% a4=single(1);
% end
% %%%%%%%%%%%%
% Ta=Tr*(a1*(jop==1)+a2*(jop==2));
% Tb=Tr*(a3*(jop==1)+a4*(jop==2));

% Ta=Tr*((jop==1));
% Tb=Tr*((jop==2));
% Ta=Tabf(jop,1);
% Tb=Tabf(jop,2);

Ta=Tao;
Tb=Tbo;


TA=(moder==1)*(Tb+Ta)+(moder==6)*(Tb+Ta)+(moder==2)*(Ta)+(moder==5)*(Tb);
TB=(moder==1)*(Tb)+(moder==2)*(Tb+Ta)+(moder==3)*(Tb+Ta)+(moder==4)*(Ta);
TC=(moder==6)*(Ta)+(moder==3)*(Tb)+(moder==4)*(Tb+Ta)+(moder==5)*(Tb+Ta);

Gates=[TA,TB,TC]';
J=jop;
Gate=Gates;

== matlab function MicroFSMPCCLACPU1/ADC-PWM /Control_System/Closed Loop Control/FS-MPC opt tiempo complex Clean 1for1 ==
  settings: updateMethod=DISCRETE
  data: I input single size=2; Gate output single size=3; FEM input single size=2; iAref input single size=1; iBref input single size=1; J output single size=1; mode input single size=1; moder input single size=1

function [Gate,J]      = fcn(I,FEM,iAref,iBref,mode,moder)


%%%%%Init Parameters%%%%%%%
Ts=single(2.5e-5);
R=single(1) ;
L=single(2.05e-3);
M=(3/7)*L;
Ls=single(L+M);
ud=single(170);
alphe=single(0.5);
gmax=single(10000);
n=single(7);
%nk=single(3);


 persistent     Gates Gop jop  Trop Tr  status1
  if isempty(Gates)
        Gates=single([0,0,0]');
        Gop=gmax;
        jop=single(1);
        Tr=single(0);
        Trop=single(0);

% status1=[
%  1,1,0;
%  0,1,0;
%  0,0,0;]; 
     end


%%%%%%Read mesurments%%%%%%%%%%%%
iA=I(1);
iB=I(2);
eA=FEM(1);
eB=FEM(2);


%%%%Moded
%  if mode==1
%  status1=[0,0,0;
%  1,0,0	;
% 1,1,0;];   
%  u1=ud*[0	,	0	;
% 2/3	,	0	;
% 1/3	,	1/sqrt(3)];
% elseif mode==2
%  status1=[0,0,0;
% 1,1,0	;
% 0,1,0	;];   
%  u1=ud*[0	,	0	;
% 1/3	,	1/sqrt(3)	;
% -1/3	,	1/sqrt(3)	;];   
% elseif mode==3
%  status1=[0,0,0;
% 0,1,0	;
% 0,1,1	;];   
%  u1=ud*[0	,	0	;
% -1/3	,	1/sqrt(3)	;
% -2/3	,	0	;];  
%  elseif mode==4
%  status1=[0,0,0;
%  0,1,1	;
% 0,0,1	;];   
%  u1=ud*[0	,	0	;
% -2/3	,	0	;
% -1/3	,	-1/sqrt(3)	;];
%  elseif mode==5
%  status1=[0,0,0;
%  0,0,1	;
% 1,0,1	;];   
%  u1=ud*[0	,	0	;
% -1/3	,	-1/sqrt(3)	;
% 1/3	,	-1/sqrt(3)	;];
%  elseif mode==6
%  status1=[0,0,0
% 1,0,1	;
%  1,0,0	;];   
%  u1=ud*[0	,	0	;
% 1/3	,	-1/sqrt(3)	;
% 2/3	,	0	;];
% 
% else
%  status1=[0,0,0;
%  1,0,0	;
% 1,1,0;];   
%  u1=ud*[0	,	0	;
% 2/3	,	0	;
% 1/3	,	1/sqrt(3)]; 
% end

%%%13 vectores totales, 12 modes
 if mode==1 %%%%V0,V1,V12
 u1=ud*[2/3	,	0	;
1/2	,	1/(2*sqrt(3));
0	,	0	;];
elseif mode==2 %%%%V0,V12,V2
 u1=ud*[1/2	,	1/(2*sqrt(3))	;
1/3	,	1/sqrt(3);
0	,	0	;];

elseif mode==3
  u1=ud*[1/3	,	1/sqrt(3)	;
0	,	1/sqrt(3)	;
0	,	0	;];   
  elseif mode==4
  u1=ud*[0	,	1/sqrt(3)	;
-1/3	,	1/sqrt(3)	;
0	,	0	;]; 


elseif mode==5
 u1=ud*[-1/3	,	1/sqrt(3)	;
-1/2	,	1/(2*sqrt(3))	;
0	,	0	;];  

elseif mode==6
 u1=ud*[-1/2	,	1/(2*sqrt(3))	;
-2/3	,	0	;
0	,	0	;];  

 elseif mode==7
 u1=ud*[-2/3	,	0	;
-1/2	,	-1/(2*sqrt(3));
0	,	0	;];

  elseif mode==8
 u1=ud*[-1/2	,	-1/(2*sqrt(3))	;
-1/3	,	-1/sqrt(3)	;
0	,	0	;];


 elseif mode==9
 u1=ud*[
-1/3	,	-1/sqrt(3)	;
0	,	-1/sqrt(3)	;
0	,	0	;];

  elseif mode==10
 u1=ud*[
0	,	-1/sqrt(3)	;
1/3	,	-1/sqrt(3)	;
0	,	0	;];


 elseif mode==11
 u1=ud*[
1/3	,	-1/sqrt(3)	;
1/2	,	-1/(2*sqrt(3))	;
0	,	0	;];

  elseif mode==12
 u1=ud*[
1/2	,	-1/(2*sqrt(3))	;
2/3	,	0	;
0	,	0	;];

else
 
 u1=ud*[
2/3	,	0	;
1/3	,	1/sqrt(3);
0	,	0	;]; 
end
%%%%%%%%FSMPC%%%%%%%%%%%%%%%%%%%%%%%%%%%%%%%%%%%%%

      Gop=gmax;
      jop=single(1);
       ar=single(0.9/7);
%%%%%%For n loop N1  %%%%%% 
% for p= 1:nk
% 
%     if p==1
%         n=single(3);
%     else
%         n=single(2);
%     end    
%     Tr1=ar*(2*p);

%%%%%%%%%%%%%%%%%%%%%%%%%%%%%%%%%%%%%%%%%%%%%%%%%%
     for j= 1:n    

% switch j
%     case 1
%         Tr1=ar*single(2);
%         v=single(1);
%     case 2
%         Tr1=ar*single(2);
%         v=single(2);
%      case 3
%         Tr1=ar*single(2);
%         v=single(3) ; 
% 
%     case 4
%         Tr1=ar*single(4);
%         v=single(1);
%     case 5
%         Tr1=ar*single(4);
%         v=single(2);
%     case 6
%         Tr1=ar*single(6);
%         v=single(1);     
%     case 7
%         Tr1=ar*single(6);
%         v=single(2) ; 
%        
%     otherwise
%         Tr1=ar*single(2);
%         v=single(1);
% end

if j<=7
v=single(2-mod(j,2));
else
v=single(3);
end
if j<=2
    Tr1=ar*single(2);
elseif j<=4
  Tr1=ar*single(4);
else
     Tr1=ar*single(6);
end



     uA1=u1((v),1);
     uB1=u1((v),2);
%%%%%%For loop %%%%%%%%%%%%%%%%%%%%%%%%%%%%%%%%% 
%      iA1= iA + (1/Ls)*(Tr1*Ts*uA1)- (Ts/Ls)*(eA+R*iA);
%      iB1=iB + (1/Ls)*(Tr1*Ts*uB1)- (Ts/Ls)*(eB+R*iB);
     iA1= (1/(Ts*R+Ls))*(Ls*iA+(Tr1*Ts*uA1)- Ts*eA);
     iB1=(1/(Ts*R+Ls))*(Ls*iB+(Tr1*Ts*uB1)- Ts*eB);
     G=(iAref-iA1)^2+(iBref-iB1)^2 ; 
     % G=abs(iAref-iA1)+abs(iBref-iB1) ; 
          if G<Gop
          Gop=G;
          jop=v;
          Tr=Tr1;
          end
     end
%end
%%%%%%%%%%%%%%%%%%%%%%%%%%%%%%%%%%%%%%%%%%%%%%%%%

% %%%%Segunda vuelta%%%%%
%      uA1=u1((jop),1);
%      uB1=u1((jop),2);
% %%%%%%%%%%%%%%%%%%%%%%%%%%%%%%%%%%%%%%%%%%%%%%%%%%
% %      for p= 1:2    
% % %%%%%%For loop %%%%%%%%%%%%%%%%%%%%%%%%%%%%%%%%% 
% %     if p==1
% %      Trop=Tr;
% %      Tr1=Trop-ar; 
% %      else
% %      Tr1=Trop+ar;
% %     end
%   for j= 1:2 
%      if j==1
%      Trop=Tr;
%      Tr1=Trop-ar; 
%      else
%      Tr1=Trop+ar;
%     end
% %      uA1=u1((j),1);
% %      uB1=u1((j),2);
%      iA1= iA + (1/Ls)*(Tr1*Ts*uA1)- (Ts/Ls)*(eA+R*iA);
%      iB1=iB + (1/Ls)*(Tr1*Ts*uB1)- (Ts/Ls)*(eB+R*iB);
%      G=(iAref-iA1)^2+(iBref-iB1)^2 ; 
%        %G=abs(iAref-iA1)+abs(iBref-iB1) ; 
%           if G<Gop
%           Gop=G;
%           Tr=Tr1;
%           end
%   end
   %  end

%%%%%%%%%%%%%%%%%%%%%%%%%%%%%%%%%%%%%%%%%%%%%%%%%
    
%%%%Apply conmutation states%%%%%%%%%%%%%%%%%%%%%%%  


%%%%%%12 vectores
if mod(mode,2)==1
a1=single(1);
a2=alphe;
a3=single(0);
a4=alphe;
else
a1=alphe;
a2=single(0);
a3=alphe;
a4=single(1);
end
% %%%%%%%%%%%%
Ta=Tr*(a1*(jop==1)+a2*(jop==2));
Tb=Tr*(a3*(jop==1)+a4*(jop==2));

% Ta=Tr*((jop==1));
% Tb=Tr*((jop==2));


TA=(moder==1)*(Tb+Ta)+(moder==6)*(Tb+Ta)+(moder==2)*(Ta)+(moder==5)*(Tb);
  TB=(moder==1)*(Tb)+(moder==2)*(Tb+Ta)+(moder==3)*(Tb+Ta)+(moder==4)*(Ta);
  TC=(moder==6)*(Ta)+(moder==3)*(Tb)+(moder==4)*(Tb+Ta)+(moder==5)*(Tb+Ta);

Gates=[TA,TB,TC]';
J=jop;
Gate=Gates;

== matlab function MicroFSMPCCLACPU1/ADC-PWM /Control_System/Closed Loop Control/FS-MPC opt tiempo complex Clean 1for2 ==
  settings: updateMethod=DISCRETE
  data: I input single size=2; Gate output single size=3; FEM input single size=2; iAref input single size=1; iBref input single size=1; J output single size=1; mode input single size=1

function [Gate,J]      = fcn(I,FEM,iAref,iBref,mode)


%%%%%Init Parameters%%%%%%%
%Ts=single(5e-5);
Ts=single(3.2e-5);
R=single(1) ;
L=single(2.02e-3);
%L=single(Lp);
M=(3/7)*L;
Ls=single(L+M);
ud=single(170);
%alphe=single(0.5);
gmax=single(10000);
n=single(7);
%nk=single(3);
moder=mode;

 persistent     Gates Gop jop  Trop Tr  status1
  if isempty(Gates)
        Gates=single([0,0,0]');
        Gop=gmax;
        jop=single(1);
        Tr=single(0);
        Trop=single(0);

% status1=[
%  1,1,0;
%  0,1,0;
%  0,0,0;]; 
     end


%%%%%%Read mesurments%%%%%%%%%%%%
iA=I(1);
iB=I(2);
eA=FEM(1);
eB=FEM(2);


%%%%Moded
%  if mode==1
%  status1=[0,0,0;
%  1,0,0	;
% 1,1,0;];   
%  u1=ud*[0	,	0	;
% 2/3	,	0	;
% 1/3	,	1/sqrt(3)];
% elseif mode==2
%  status1=[0,0,0;
% 1,1,0	;
% 0,1,0	;];   
%  u1=ud*[0	,	0	;
% 1/3	,	1/sqrt(3)	;
% -1/3	,	1/sqrt(3)	;];   
% elseif mode==3
%  status1=[0,0,0;
% 0,1,0	;
% 0,1,1	;];   
%  u1=ud*[0	,	0	;
% -1/3	,	1/sqrt(3)	;
% -2/3	,	0	;];  
%  elseif mode==4
%  status1=[0,0,0;
%  0,1,1	;
% 0,0,1	;];   
%  u1=ud*[0	,	0	;
% -2/3	,	0	;
% -1/3	,	-1/sqrt(3)	;];
%  elseif mode==5
%  status1=[0,0,0;
%  0,0,1	;
% 1,0,1	;];   
%  u1=ud*[0	,	0	;
% -1/3	,	-1/sqrt(3)	;
% 1/3	,	-1/sqrt(3)	;];
%  elseif mode==6
%  status1=[0,0,0
% 1,0,1	;
%  1,0,0	;];   
%  u1=ud*[0	,	0	;
% 1/3	,	-1/sqrt(3)	;
% 2/3	,	0	;];
% 
% else
%  status1=[0,0,0;
%  1,0,0	;
% 1,1,0;];   
%  u1=ud*[0	,	0	;
% 2/3	,	0	;
% 1/3	,	1/sqrt(3)]; 
% end


% % %%%7 Vectores totales
 if mode==1
 u1=ud*[2/3	,	0	;
1/3	,	1/sqrt(3);
0	,	0	;];
elseif mode==2
 u1=ud*[1/3	,	1/sqrt(3)	;
-1/3	,	1/sqrt(3)	;
0	,	0	;];   
elseif mode==3
 u1=ud*[-1/3	,	1/sqrt(3)	;
-2/3	,	0	;
0	,	0	;];  
 elseif mode==4
 u1=ud*[-2/3	,	0	;
-1/3	,	-1/sqrt(3)	;
0	,	0	;];
 elseif mode==5
 u1=ud*[-1/3	,	-1/sqrt(3)	;
1/3	,	-1/sqrt(3)	;
0	,	0	;];
 elseif mode==6
 u1=ud*[1/3	,	-1/sqrt(3)	;
2/3	,	0	;
0	,	0	;];
else
 u1=ud*[2/3	,	0	;
1/3	,	1/sqrt(3);
0	,	0	;]; 
end
%%%%%%%



% %%%13 vectores totales, 12 modes
%  if mode==1 %%%%V0,V1,V12
%  u1=ud*[2/3	,	0	;
% 1/2	,	1/(2*sqrt(3));
% 0	,	0	;];
% elseif mode==2 %%%%V0,V12,V2
%  u1=ud*[1/2	,	1/(2*sqrt(3))	;
% 1/3	,	1/sqrt(3);
% 0	,	0	;];
% 
% elseif mode==3
%   u1=ud*[1/3	,	1/sqrt(3)	;
% 0	,	1/sqrt(3)	;
% 0	,	0	;];   
%   elseif mode==4
%   u1=ud*[0	,	1/sqrt(3)	;
% -1/3	,	1/sqrt(3)	;
% 0	,	0	;]; 
% 
% 
% elseif mode==5
%  u1=ud*[-1/3	,	1/sqrt(3)	;
% -1/2	,	1/(2*sqrt(3))	;
% 0	,	0	;];  
% 
% elseif mode==6
%  u1=ud*[-1/2	,	1/(2*sqrt(3))	;
% -2/3	,	0	;
% 0	,	0	;];  
% 
%  elseif mode==7
%  u1=ud*[-2/3	,	0	;
% -1/2	,	-1/(2*sqrt(3));
% 0	,	0	;];
% 
%   elseif mode==8
%  u1=ud*[-1/2	,	-1/(2*sqrt(3))	;
% -1/3	,	-1/sqrt(3)	;
% 0	,	0	;];
% 
% 
%  elseif mode==9
%  u1=ud*[
% -1/3	,	-1/sqrt(3)	;
% 0	,	-1/sqrt(3)	;
% 0	,	0	;];
% 
%   elseif mode==10
%  u1=ud*[
% 0	,	-1/sqrt(3)	;
% 1/3	,	-1/sqrt(3)	;
% 0	,	0	;];
% 
% 
%  elseif mode==11
%  u1=ud*[
% 1/3	,	-1/sqrt(3)	;
% 1/2	,	-1/(2*sqrt(3))	;
% 0	,	0	;];
% 
%   elseif mode==12
%  u1=ud*[
% 1/2	,	-1/(2*sqrt(3))	;
% 2/3	,	0	;
% 0	,	0	;];
% 
% else
%  
%  u1=ud*[
% 2/3	,	0	;
% 1/3	,	1/sqrt(3);
% 0	,	0	;]; 
% end
%%%%%%%%FSMPC%%%%%%%%%%%%%%%%%%%%%%%%%%%%%%%%%%%%%

      Gop=gmax;
      jop=single(1);
       ar=single(0.9/7);
%%%%%%For n loop N1  %%%%%% 
% for p= 1:nk
% 
%     if p==1
%         n=single(3);
%     else
%         n=single(2);
%     end    
%     Tr1=ar*(2*p);

%%%%%%%%%%%%%%%%%%%%%%%%%%%%%%%%%%%%%%%%%%%%%%%%%%
     for j= 1:n    

% switch j
%     case 1
%         Tr1=ar*single(2);
%         v=single(1);
%     case 2
%         Tr1=ar*single(2);
%         v=single(2);
%      case 3
%         Tr1=ar*single(2);
%         v=single(3) ; 
% 
%     case 4
%         Tr1=ar*single(4);
%         v=single(1);
%     case 5
%         Tr1=ar*single(4);
%         v=single(2);
%     case 6
%         Tr1=ar*single(6);
%         v=single(1);     
%     case 7
%         Tr1=ar*single(6);
%         v=single(2) ; 
%        
%     otherwise
%         Tr1=ar*single(2);
%         v=single(1);
% end

if j<=6
v=single(2-mod(j,2));
else
v=single(3);
end
if j<=2
    Tr1=ar*single(2);
elseif j<=4
  Tr1=ar*single(4);
%   elseif j<=6
%   Tr1=ar*single(6);
else
    % Tr1=ar*single(8);
      Tr1=ar*single(6);
end



     uA1=u1((v),1);
     uB1=u1((v),2);
%%%%%%For loop %%%%%%%%%%%%%%%%%%%%%%%%%%%%%%%%% 
     iA1= iA + (1/Ls)*(Tr1*Ts*uA1)- (Ts/Ls)*(eA+R*iA);
     iB1=iB + (1/Ls)*(Tr1*Ts*uB1)- (Ts/Ls)*(eB+R*iB);
%      iA1= (1/(Ts*R+Ls))*(Ls*iA+(Tr1*Ts*uA1)- Ts*eA);
%      iB1=(1/(Ts*R+Ls))*(Ls*iB+(Tr1*Ts*uB1)- Ts*eB);
     G=(iAref-iA1)^2+(iBref-iB1)^2 ; 
     % G=abs(iAref-iA1)+abs(iBref-iB1) ; 
          if G<Gop
          Gop=G;
          jop=v;
          Tr=Tr1;
          end
     end
%end
%%%%%%%%%%%%%%%%%%%%%%%%%%%%%%%%%%%%%%%%%%%%%%%%%

% %%%%Segunda vuelta%%%%%
     uA1=u1((jop),1);
     uB1=u1((jop),2);
% %%%%%%%%%%%%%%%%%%%%%%%%%%%%%%%%%%%%%%%%%%%%%%%%%%
% %      for p= 1:2    
% % %%%%%%For loop %%%%%%%%%%%%%%%%%%%%%%%%%%%%%%%%% 
% %     if p==1
% %      Trop=Tr;
% %      Tr1=Trop-ar; 
% %      else
% %      Tr1=Trop+ar;
% %     end
  for j= 1:2 
     if j==1
     Trop=Tr;
     Tr1=Trop-ar; 
     else
     Tr1=Trop+ar;
    end
%      uA1=u1((j),1);
%      uB1=u1((j),2);
     iA1= iA + (1/Ls)*(Tr1*Ts*uA1)- (Ts/Ls)*(eA+R*iA);
     iB1=iB + (1/Ls)*(Tr1*Ts*uB1)- (Ts/Ls)*(eB+R*iB);
     G=(iAref-iA1)^2+(iBref-iB1)^2 ; 
       %G=abs(iAref-iA1)+abs(iBref-iB1) ; 
          if G<Gop
          Gop=G;
          Tr=Tr1;
          end
  end
 %   end

%%%%%%%%%%%%%%%%%%%%%%%%%%%%%%%%%%%%%%%%%%%%%%%%%
    
%%%%Apply conmutation states%%%%%%%%%%%%%%%%%%%%%%%  


%%%%%%12 vectores
% if mod(mode,2)==1
% a1=single(1);
% a2=alphe;
% a3=single(0);
% a4=alphe;
% else
% a1=alphe;
% a2=single(0);
% a3=alphe;
% a4=single(1);
% end
% %%%%%%%%%%%%
% Ta=Tr*(a1*(jop==1)+a2*(jop==2));
% Tb=Tr*(a3*(jop==1)+a4*(jop==2));

Ta=Tr*((jop==1));
Tb=Tr*((jop==2));


TA=(moder==1)*(Tb+Ta)+(moder==6)*(Tb+Ta)+(moder==2)*(Ta)+(moder==5)*(Tb);
TB=(moder==1)*(Tb)+(moder==2)*(Tb+Ta)+(moder==3)*(Tb+Ta)+(moder==4)*(Ta);
TC=(moder==6)*(Ta)+(moder==3)*(Tb)+(moder==4)*(Tb+Ta)+(moder==5)*(Tb+Ta);

Gates=[TA,TB,TC]';
J=jop;
Gate=Gates;

== matlab function MicroFSMPCCLACPU1/ADC-PWM /Control_System/Closed Loop Control/Power Trayectory ==
  settings: updateMethod=DISCRETE
  data: Pref input; P output; th input; Q output; moder output
function [P,Q,moder]       = fcn(Pref,th)
%Kt =0.3811;
%Kt=0.3455;
%J= 0.0002618;
%Ip=single((torq)/(2*Kt));
%Ip=single(torq);
% p=single(8);
% Am =single( (6/pi));
% mph = single(pi/3);
%%%% wrap
tr = single((1)*th);
 %f = single(2*pi);
%tr =single( mod(the,f));
% i_A = single(0); i_B = single(0); i_C =single(0);
 mode=single(0);


%%%%%%%%%Hexagono
% if(0<=tr && tr<=pi/3)
%     i_A = single(-3*tr*sqrt(3)/(2*pi));
%      i_B = single(-3*tr/(2*pi) +1);
% 
%        elseif(pi/3<tr && tr<2*pi/3)
%     i_A = single(-sqrt(3)/(2));
%      i_B = single(-3*tr/(pi)+1.5);
% 
%        elseif(2*pi/3<tr && tr<pi)
%     i_A =single( 3*tr*sqrt(3)/(2*pi)-3*sqrt(3)/(2));
%      i_B = single(-3*tr/(2*pi) +1/2);
% 
%        elseif(pi<tr && tr<4*pi/3)
%     i_A =single( 3*tr*sqrt(3)/(2*pi)-3*sqrt(3)/(2));
%      i_B = single(3*tr/(2*pi) -5/2);
% 
%         elseif(4*pi/3<tr && tr<5*pi/3)
%       i_A = single(sqrt(3)/(2));
%      i_B =single( 3*tr/(pi)-4.5);
% 
%         elseif(5*pi/3<tr && tr<6*pi/3)
%           i_A =single( -3*tr*sqrt(3)/(2*pi)+3*sqrt(3));
%      i_B = single(3*tr/(2*pi) -2);
%  
% else
%          i_A = single(0);
% end



%%%%%%%%%
%%%% e_A
% 
% if(0<=tr && tr<=pi/6)
%     i_A = single(0);
% elseif((pi)/6<tr && tr<=5*pi/6)
%     i_A = single(-1);
%   elseif(5*pi/6<tr && tr<=(7*pi)/6)
%         i_A =single( 0);
%     elseif((7*pi)/6<tr && tr<11*pi/6)
%         i_A = single(1);
%           elseif((11*pi)/6<tr && tr<12*pi/6)
%         i_A =single(0);
% end
% %%%% i_B
% if(0<=tr && tr<=pi/2)
%     i_B = single(1);
% elseif(pi/2<tr && tr<=(5*pi)/6)
%     i_B = single(0);
% elseif((5*pi)/6<tr && tr<=(3*pi)/2)
%     i_B = single(-1);
%   elseif((3*pi)/2<tr && tr<=(11*pi)/6)
%         i_B =single(0);
%     elseif((11*pi)/6<tr && tr<2*pi)
%         i_B = single(1);
% end
% %%%% i_C
% if(0<=tr && tr<=pi/6)
%     i_C = single(-1);
% elseif(pi/6<tr && tr<=(pi)/2)
%     i_C =single( 0);
% elseif((pi)/2<tr && tr<=(7*pi)/6)
%     i_C = single(1);
%   elseif((7*pi)/6<tr && tr<=(3*pi)/2)
%         i_C = single(0);
%     elseif((3*pi)/2<tr && tr<2*pi)
%         i_C = single(-1);
% end
%%%mode
% 
% if(0<=tr && tr<pi/3)
%     mode=1;
% elseif(pi/3<=tr && tr<(2*pi)/3)
%       mode=2;
% elseif((2*pi)/3<=tr && tr<pi)
%     mode=3;
%   elseif(pi<=tr && tr<(4*pi)/3)
%           mode=4;
%     elseif((4*pi)/3<=tr && tr<(5*pi)/3)
%          mode=5;     
%     elseif((5*pi)/3<=tr && tr<2*pi)
%         mode=6;
% end
% 
% 
% if(0<=tr && tr<pi/3)
%     mode=single(1);
% elseif(pi/3<=tr && tr<(2*pi)/3)
%       mode=single(2);
% elseif((2*pi)/3<=tr && tr<pi)
%     mode=single(3);
%   elseif(pi<=tr && tr<(4*pi)/3)
%           mode=single(4);
%     elseif((4*pi)/3<=tr && tr<(5*pi)/3)
%          mode=single(5);     
%     elseif((5*pi)/3<=tr && tr<(6*pi)/3)
%         mode=single(6);
%  end
% moder=single(mode);
% 
% 
if(0<=tr && tr<pi/6)
    mode=single(2);
elseif(pi/6<=tr && tr<(3*pi)/6)
      mode=single(3);
elseif((3*pi)/6<=tr && tr<(5*pi)/6)
    mode=single(4);
  elseif((5*pi)/6<=tr && tr<(7*pi)/6)
          mode=single(5);
    elseif((7*pi)/6<=tr && tr<(9*pi)/6)
         mode=single(6);     
    elseif((9*pi)/6<=tr && tr<(11*pi)/6)
        mode=single(1);
        elseif((11*pi)/6<=tr && tr<(12*pi)/6)
        mode=single(2);
end
moder=single(mode);
%%%%%
% Ira=single(Ip*i_A);
% Irb=single(Ip*i_B);
% Irc=single(Ip*i_C);
% % Ia=Ira;
% Ia=single((2/3)*(Ira-(1/2)*(Irb)-(1/2)*Irc));
% Ib=single((2/3)*((sqrt(3)/2)*(Irb)-(sqrt(3)/2)*Irc));

% Ia=Ip*2/sqrt(3)*i_A;
% Ib=Ip*2/sqrt(3)*i_B;
P=Pref;
Q=single(0);
%%%%%

== matlab function MicroFSMPCCLACPU1/ADC-PWM /Control_System/Closed Loop Control/Trajectory ==
  settings: updateMethod=DISCRETE
  data: torq input; Ia output; th input; Ib output; moder output
function [Ia,Ib,moder]       = fcn(torq,th)
% Kt=0.3455;
% J= 0.0002618;
%Ip=single((J*torq)/(2*Kt));
Ip=single(torq);
p=single(8);
Am =single( (6/pi));
mph = single(pi/3);
%%%% wrap
tr = single((1)*th);
 %f = single(2*pi);
%tr =single( mod(the,f));
i_A = single(0); i_B = single(0); i_C =single(0);
mode=single(0)
%%%% e_A
%%
if(0<=tr && tr<=pi/3)
    i_A = single(-3*tr*sqrt(3)/(2*pi));
     i_B = single(-3*tr/(2*pi) +1);

       elseif(pi/3<tr && tr<2*pi/3)
    i_A = single(-sqrt(3)/(2));
     i_B = single(-3*tr/(pi)+1.5);

       elseif(2*pi/3<tr && tr<pi)
    i_A =single( 3*tr*sqrt(3)/(2*pi)-3*sqrt(3)/(2));
     i_B = single(-3*tr/(2*pi) +1/2);

       elseif(pi<tr && tr<4*pi/3)
    i_A =single( 3*tr*sqrt(3)/(2*pi)-3*sqrt(3)/(2));
     i_B = single(3*tr/(2*pi) -5/2);

        elseif(4*pi/3<tr && tr<5*pi/3)
      i_A = single(sqrt(3)/(2));
     i_B =single( 3*tr/(pi)-4.5);

        elseif(5*pi/3<tr && tr<6*pi/3)
          i_A =single( -3*tr*sqrt(3)/(2*pi)+3*sqrt(3));
     i_B = single(3*tr/(2*pi) -2);
 
else
         i_A = single(0);
end

%%%mode
% 
% if(0<=tr && tr<pi/3)
%     mode=1;
% elseif(pi/3<=tr && tr<(2*pi)/3)
%       mode=2;
% elseif((2*pi)/3<=tr && tr<pi)
%     mode=3;
%   elseif(pi<=tr && tr<(4*pi)/3)
%           mode=4;
%     elseif((4*pi)/3<=tr && tr<(5*pi)/3)
%          mode=5;     
%     elseif((5*pi)/3<=tr && tr<2*pi)
%         mode=6;
% end
% 

% if(0<=tr && tr<pi/3)
%     mode=single(1);
% elseif(pi/3<=tr && tr<(2*pi)/3)
%       mode=single(2);
% elseif((2*pi)/3<=tr && tr<pi)
%     mode=single(3);
%   elseif(pi<=tr && tr<(4*pi)/3)
%           mode=single(4);
%     elseif((4*pi)/3<=tr && tr<(5*pi)/3)
%          mode=single(5);     
%     elseif((5*pi)/3<=tr && tr<(6*pi)/3)
%         mode=single(6);
%  end
% moder=single(mode);

if(0<=tr && tr<pi/6)
    mode=single(2);
elseif(pi/6<=tr && tr<(3*pi)/6)
      mode=single(3);
elseif((3*pi)/6<=tr && tr<(5*pi)/6)
    mode=single(4);
  elseif((5*pi)/6<=tr && tr<(7*pi)/6)
          mode=single(5);
    elseif((7*pi)/6<=tr && tr<(9*pi)/6)
         mode=single(6);     
    elseif((9*pi)/6<=tr && tr<(11*pi)/6)
        mode=single(1);
        elseif((11*pi)/6<=tr && tr<(12*pi)/6)
        mode=single(2);
end
moder=single(mode);

%%%%%

Ia=single(Ip*2/sqrt(3)*i_A);
Ib=single(Ip*2/sqrt(3)*i_B);
%%%%%
